simulink model "Simulink_Observation_5"  (R2020b)
settings: Solver=VariableStepAuto  StartTime=0.0  StopTime=39  RelTol=1e-3
libraries: dspsnks4 x1, dspvision x1
settings Model: Creator=Mohit Akhouri  LastModifiedBy=Mohit Akhouri

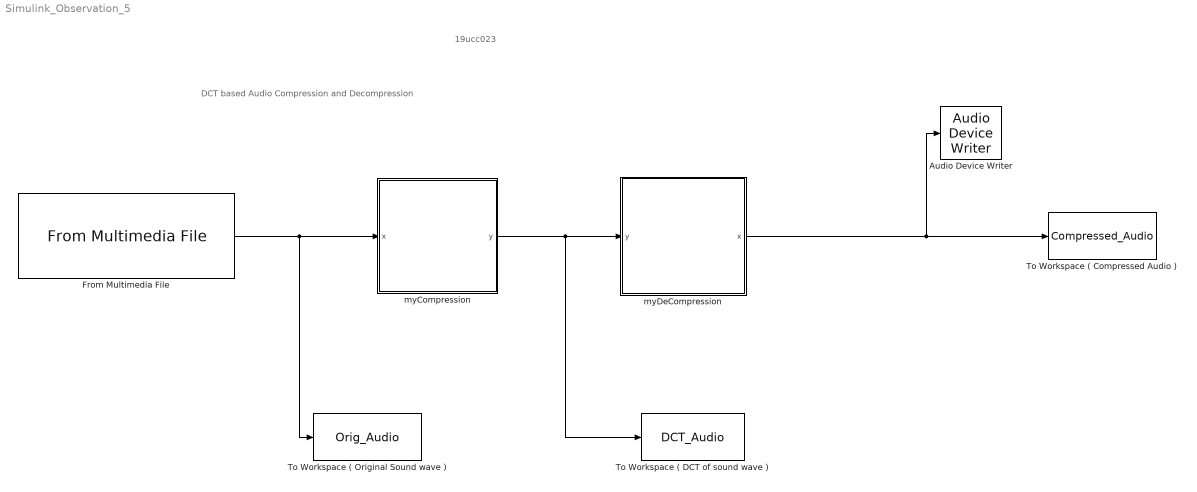
== system Simulink_Observation_5 ==
  note: DCT based Audio Compression and Decompression
  note: 19ucc023
  Audio Device Writer : dspsnks4/Audio Device Writer  Driver=DirectSound  Device=Default  InheritSampleRate=on  SampleRate=44100  BitDepth=16-bit integer  BufferSize=4096  NumBuffers=10  DefaultOutputChannelMapping=on  OutputChannelMapping=1:2  OutputNumUnderrunSamples=off  DriverIdx=1  DeviceWarnFlag=''
  From Multimedia File : dspvision/From Multimedia File  inputFilename=C:\Users\Mohit Akhouri\Desktop\DSP_LAB_EXP_7\input.wav  readRange=[1 Inf]  loop=on  numPlays=inf  outputStreams=Audio only  videoDataType=single  audioDataType=double  inheritSampleTime=on  userDefinedSampleTime=1/30  noAudioOutput=off  isIntensityVideo=off  fourcc=RGB  colorVideoFormat=Separate color signals  outputEOF=off  dataOrg=Column-major  audioFrameSize=1024  computeAudioFrameSize=off  outSamplingMode=Sample based
  To Workspace ( Compressed Audio ) : ToWorkspace  VariableName=Compressed_Audio  SaveFormat=Timeseries  SampleTime=-1
  To Workspace ( DCT of sound wave ) : ToWorkspace  VariableName=DCT_Audio  SaveFormat=Timeseries  SampleTime=-1
  To Workspace ( Original Sound wave ) : ToWorkspace  VariableName=Orig_Audio  SaveFormat=Timeseries  SampleTime=-1
  myCompression : MATLAB Function  TreatAsAtomicUnit=on
  myDeCompression : MATLAB Function  TreatAsAtomicUnit=on
  wires:
  From Multimedia File/1 -> To Workspace ( Original Sound wave )/1, myCompression/1(x)
  myCompression/1(y) -> To Workspace ( DCT of sound wave )/1, myDeCompression/1(y)
  myDeCompression/1(x) -> Audio Device Writer/1, To Workspace ( Compressed Audio )/1

== matlab function Simulink_Observation_5/myDeCompression ==
  data: y input; x output
function x = fcn(y)

% 19ucc023
% Mohit Akhouri

% This function will perform DeCompression of audio signal

x = idct(y);

== matlab function Simulink_Observation_5/myCompression ==
  data: x input; y output
function y = fcn(x)

% 19ucc023
% Mohit Akhouri

% This function will perform Compression of audio signal 'input.wav'
[x1,fs] = audioread('input.wav');
y = dct(x1);
